simulink model "QD2_MissionCtrl_Swarm_4x_R2021a"  (R2021a)
settings: Solver=ode2  StartTime=0.0  StopTime=inf  FixedStep=0.001  RelTol=1e-3  EnableMultiTasking=on
undefined symbols (not defined in the file): datetime, Host, localhost, m, qc_get_step_size, saved_data
libraries: quarc_library x48, simulink x13, simulink_extras x1
(part 1 of 2)
settings Model: SimulationMode=external  ExtModeTrigDuration=10000  Creator=Admin  LastModifiedBy=jpineros
settings SolverCC: AlgebraicLoopSolver=TrustRegion  PositivePriorityOrder=on
settings DataIOCC: ReturnWorkspaceOutputs=off
settings DebuggingCC: SFUnexpectedBacktrackingDiag=warning  SFNoUnconditionalDefaultTransitionDiag=warning  SFExecutionAtInitializationDiag=none  ArithmeticOperatorsInVariantConditions=warning
settings SFSimCC: SimUseLocalCustomCode=off  CustomCodeUndefinedFunction=UseInterfaceOnly
settings RTWCC: Description=QUARC Win64 Target Using Toolchain  SystemTargetFile=quarc_win64.tlc  TemplateMakefile=quarc_default_tmf  RTWUseLocalCustomCode=off  Toolchain=QUARC win64 | nmake (64-bit Windows)  BuildConfiguration=Faster Runs  DLArmComputeVersion=20.02.1
settings CodeAppCC: StateflowObjectComments=on
settings STFCustomTargetCC: ConcurrentExecutionCompliant=on  SystemTargetFile=quarc_win64.tlc
settings GRTTargetCC: TargetLangStandard=C89/C90 (ANSI)  ParMdlRefBuildCompliant=off  CompOptLevelCompliant=off  CombineOutputUpdateFcns=off  MatFileLogging=off  CPPClassGenCompliant=off  GRTInterface=on  ExtMode=on  ExtModeMexFile=quarc_comm  ExtModeMexArgs='-w -d %d -uri %u -URI_Host_V1 tcpip://localhost:18001 -URI_Host_V2 tcpip://localhost:18002 -URI_Host_V3 tcpip://localhost:18003 -URI_Host_V4 tcpip://localhost:18004'
settings ConfigComp: CovMetricSettings=dw  CovSaveCumulativeToWorkspaceVar=on  CovSaveSingleToWorkspaceVar=on  CovExternalEMLEnable=off

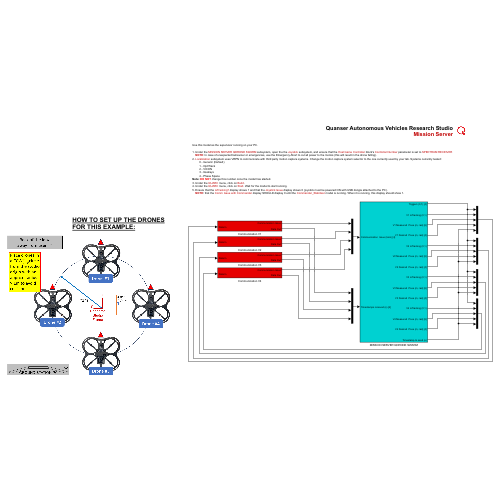
[thumbnail: Simulink's stored preview of the top-level diagram]
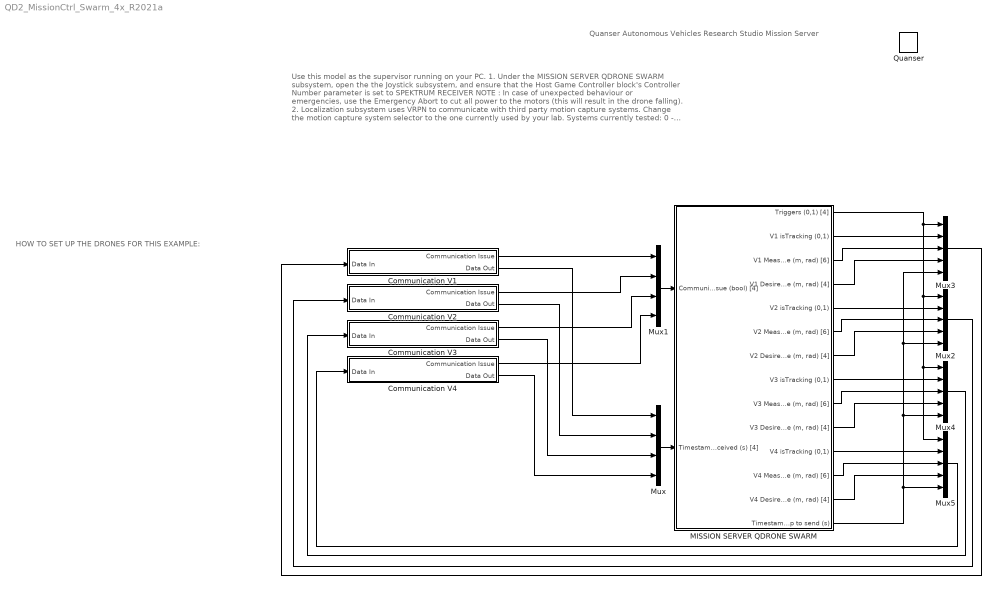
== system QD2_MissionCtrl_Swarm_4x_R2021a ==
  note: Use this model as the supervisor running on your PC.
      |
      | 1. Under the MISSION SERVER QDRONE SWARM subsystem, open the the Joystick subsystem, and ensure that the Host Game Controller block's Controller Number parameter is set to SPEKTRUM RECEIVER
      | NOTE : In case of unexpected behaviour or emergencies, use the Emergency Abort to cut all power to the motors (this will result in the drone falling).
      | 2. Localization subsystem uses VRPN to communicate with third party motion capture systems. Change the motion capture system selector to the one currently used by your lab. Systems currently tested:
      | 0 - Generic (Default)
      | 1 - OptiTrack
      | 2 - VICON
      | 3 - Qualisys
      | 4 - Phase Space
      | Note: DO NOT change this number once the model has started.
      | 3. Under the QUARC menu, click on Build .
      | 4. Under the QUARC menu, click on Start . Wait for the model to start running.
      | 5. Ensure that the isTracking? display shows 1 and that the Joystick Issue display shows 0 (joystick must be powered ON with USB dongle attached to the PC).
      | NOTE : that the Comm Issue with Commander display SHOULD display 0 until the Commander_Stabilizer model is running. When it is running, this display should show 1.
  note: Quanser Autonomous Vehicles Research Studio
      | Mission Server
  note: HOW TO SET UP THE DRONES FOR THIS EXAMPLE:
  Communication V1 : Subsystem
  Communication V2 : Subsystem
  Communication V3 : Subsystem
  Communication V4 : Subsystem
  MISSION SERVER QDRONE SWARM : Subsystem
  Mux : Mux
  Mux1 : Mux
  Mux{2..5} (4 alike) : Mux  Inputs=5
  Quanser : quarc_library/Logos/Quanser
  wires:
  Communication V1/1(Communication Issue) -> Mux1/1
  Communication V2/1(Communication Issue) -> Mux1/2
  Communication V3/1(Communication Issue) -> Mux1/3
  Communication V4/1(Communication Issue) -> Mux1/4
  Communication V4/2(Data Out) -> Mux/4
  Communication V3/2(Data Out) -> Mux/3
  Communication V2/2(Data Out) -> Mux/2
  Communication V1/2(Data Out) -> Mux/1
  MISSION SERVER QDRONE SWARM/14(Timestamp to send (s)) -> Mux5/5, Mux3/5, Mux2/5, Mux4/5
  Mux3/1 -> Communication V1/1(Data In)
  Mux2/1 -> Communication V2/1(Data In)
  Mux4/1 -> Communication V3/1(Data In)
  Mux5/1 -> Communication V4/1(Data In)
  Mux1/1 -> MISSION SERVER QDRONE SWARM/1(Communication Issue (bool) [4])
  Mux/1 -> MISSION SERVER QDRONE SWARM/2(Timestamps received (s) [4])
  MISSION SERVER QDRONE SWARM/3("V1 Measured Pose (m, rad) [6]") -> Mux3/3
  MISSION SERVER QDRONE SWARM/4("V1 Desired Pose (m, rad) [4]") -> Mux3/4
  MISSION SERVER QDRONE SWARM/6("V2 Measured Pose (m, rad) [6]") -> Mux2/3
  MISSION SERVER QDRONE SWARM/7("V2 Desired Pose (m, rad) [4]") -> Mux2/4
  MISSION SERVER QDRONE SWARM/9("V3 Measured Pose (m, rad) [6]") -> Mux4/3
  MISSION SERVER QDRONE SWARM/10("V3 Desired Pose (m, rad) [4]") -> Mux4/4
  MISSION SERVER QDRONE SWARM/12("V4 Measured Pose (m, rad) [6]") -> Mux5/3
  MISSION SERVER QDRONE SWARM/13("V4 Desired Pose (m, rad) [4]") -> Mux5/4
  MISSION SERVER QDRONE SWARM/1(Triggers (0,1) [4]) -> Mux5/1, Mux4/1, Mux2/1, Mux3/1
  MISSION SERVER QDRONE SWARM/2(V1 isTracking (0,1)) -> Mux3/2
  MISSION SERVER QDRONE SWARM/5(V2 isTracking (0,1)) -> Mux2/2
  MISSION SERVER QDRONE SWARM/8(V3 isTracking (0,1)) -> Mux4/2
  MISSION SERVER QDRONE SWARM/11(V4 isTracking (0,1)) -> Mux5/2

== system QD2_MissionCtrl_Swarm_4x_R2021a/Communication V1 ==
  note: Argument (-URI_Host_V1) is set at the MEX-file arguments
      | found at Model Configuration Properties > Code Generation > Interface
      |
      | Format:
      | tcpip://localhost:18001
  Data In : Inport
  Constant : Constant
  Detect Communication loss : Subsystem
  Model Argument : quarc_library/Sources/Signals/Model Argument  argument_name=URI_Host_V1  has_value=on  data_type_mode=Specify via dialog  data_type=char  max_length=80  default_value=0  default_string=tcpip://localhost:18001  variable_size=off
      settings: AttributesFormatString=(-%<argument_name>)  SourceProductName=QUARC Targets
  Stream Server : quarc_library/Communications/Basic/Stream Server  uri_source=External input port  uri=tcpip://localhost:18877  send_buffer_size=1460  receive_buffer_size=1460  byte_order=little endian (Intel - LSB first)  optimization=Minimum latency  send_options=Send most recent data  receive_options=Receive most recent data  default_value=zeros(1,1)  sample_time=qc_get_step_size  active=off  implementation=Use blocking I/O in a separate thread  send_fifo_size=1000  receive_fifo_size=1000  send_priority=0  receive_priority=0  send_dimensions=off  receive_dimensions=off  max_dimensions=-1  data_type=Inherited via back propagation  type_expr=BusObject
  "String Display " : quarc_library/Strings/String Display  alignment=center  display_mode=Single line  sample_time=-1  use_new=off
      settings: SourceProductName=QUARC Targets
  Terminator1 : Terminator
  Terminator2 : Terminator
  Communication Issue : Outport  VectorParamsAs1DForOutWhenUnconnected=off
  Data Out : Outport  Port=2  VectorParamsAs1DForOutWhenUnconnected=off
  wires:
  Detect Communication loss/1(Communication Issue (0,1)) -> Communication Issue/1
  Stream Server/1 -> Detect Communication loss/1(State)
  Stream Server/2 -> Detect Communication loss/2(Error)
  Stream Server/4 -> Data Out/1
  Model Argument/1 -> Stream Server/3, "String Display "/1
  Stream Server/5 -> Terminator1/1
  Stream Server/3 -> Terminator2/1
  Data In/1 -> Stream Server/1
  Constant/1 -> Stream Server/2

== system QD2_MissionCtrl_Swarm_4x_R2021a/Communication V2 ==
  note: Argument (-URI_Host_V2) is set at the MEX-file arguments
      | found at Model Configuration Properties > Code Generation > Interface
      |
      | Format:
      | tcpip://localhost:18002
  Data In : Inport
  Constant : Constant
  Detect Communication loss : Subsystem
  Model Argument : quarc_library/Sources/Signals/Model Argument  argument_name=URI_Host_V2  has_value=on  data_type_mode=Specify via dialog  data_type=char  max_length=80  default_value=0  default_string=tcpip://localhost:18002  variable_size=off
      settings: AttributesFormatString=(-%<argument_name>)  SourceProductName=QUARC Targets
  Stream Server : quarc_library/Communications/Basic/Stream Server  uri_source=External input port  uri=tcpip://localhost:18877  send_buffer_size=1460  receive_buffer_size=1460  byte_order=little endian (Intel - LSB first)  optimization=Minimum latency  send_options=Send most recent data  receive_options=Receive most recent data  default_value=zeros(1,1)  sample_time=qc_get_step_size  active=off  implementation=Use blocking I/O in a separate thread  send_fifo_size=1000  receive_fifo_size=1000  send_priority=0  receive_priority=0  send_dimensions=off  receive_dimensions=off  max_dimensions=-1  data_type=Inherited via back propagation  type_expr=BusObject
  "String Display " : quarc_library/Strings/String Display  alignment=center  display_mode=Single line  sample_time=-1  use_new=off
      settings: SourceProductName=QUARC Targets
  Terminator1 : Terminator
  Terminator2 : Terminator
  Communication Issue : Outport  VectorParamsAs1DForOutWhenUnconnected=off
  Data Out : Outport  Port=2  VectorParamsAs1DForOutWhenUnconnected=off
  wires:
  Constant/1 -> Stream Server/2
  Data In/1 -> Stream Server/1
  Stream Server/3 -> Terminator2/1
  Stream Server/5 -> Terminator1/1
  Model Argument/1 -> "String Display "/1, Stream Server/3
  Stream Server/4 -> Data Out/1
  Stream Server/2 -> Detect Communication loss/2(Error)
  Stream Server/1 -> Detect Communication loss/1(State)
  Detect Communication loss/1(Communication Issue (0,1)) -> Communication Issue/1

== system QD2_MissionCtrl_Swarm_4x_R2021a/Communication V3 ==
  note: Argument (-URI_Host_V3) is set at the MEX-file arguments
      | found at Model Configuration Properties > Code Generation > Interface
      |
      | Format:
      | tcpip://localhost:18003
  Data In : Inport
  Constant : Constant
  Detect Communication loss : Subsystem
  Model Argument : quarc_library/Sources/Signals/Model Argument  argument_name=URI_Host_V3  has_value=on  data_type_mode=Specify via dialog  data_type=char  max_length=80  default_value=0  default_string=tcpip://localhost:18003  variable_size=off
      settings: AttributesFormatString=(-%<argument_name>)  SourceProductName=QUARC Targets
  Stream Server : quarc_library/Communications/Basic/Stream Server  uri_source=External input port  uri=tcpip://localhost:18877  send_buffer_size=1460  receive_buffer_size=1460  byte_order=little endian (Intel - LSB first)  optimization=Minimum latency  send_options=Send most recent data  receive_options=Receive most recent data  default_value=zeros(1,1)  sample_time=qc_get_step_size  active=off  implementation=Use blocking I/O in a separate thread  send_fifo_size=1000  receive_fifo_size=1000  send_priority=0  receive_priority=0  send_dimensions=off  receive_dimensions=off  max_dimensions=-1  data_type=Inherited via back propagation  type_expr=BusObject
  "String Display " : quarc_library/Strings/String Display  alignment=center  display_mode=Single line  sample_time=-1  use_new=off
      settings: SourceProductName=QUARC Targets
  Terminator1 : Terminator
  Terminator2 : Terminator
  Communication Issue : Outport  VectorParamsAs1DForOutWhenUnconnected=off
  Data Out : Outport  Port=2  VectorParamsAs1DForOutWhenUnconnected=off
  wires:
  Detect Communication loss/1(Communication Issue (0,1)) -> Communication Issue/1
  Stream Server/1 -> Detect Communication loss/1(State)
  Stream Server/2 -> Detect Communication loss/2(Error)
  Stream Server/4 -> Data Out/1
  Model Argument/1 -> Stream Server/3, "String Display "/1
  Stream Server/5 -> Terminator1/1
  Stream Server/3 -> Terminator2/1
  Data In/1 -> Stream Server/1
  Constant/1 -> Stream Server/2

== system QD2_MissionCtrl_Swarm_4x_R2021a/Communication V4 ==
  note: Argument (-URI_Host_V4) is set at the MEX-file arguments
      | found at Model Configuration Properties > Code Generation > Interface
      |
      | Format:
      | tcpip://localhost:18004
  Data In : Inport
  Constant : Constant
  Detect Communication loss : Subsystem
  Model Argument : quarc_library/Sources/Signals/Model Argument  argument_name=URI_Host_V4  has_value=on  data_type_mode=Specify via dialog  data_type=char  max_length=80  default_value=0  default_string=tcpip://localhost:18004  variable_size=off
      settings: AttributesFormatString=(-%<argument_name>)  SourceProductName=QUARC Targets
  Stream Server : quarc_library/Communications/Basic/Stream Server  uri_source=External input port  uri=tcpip://localhost:18877  send_buffer_size=1460  receive_buffer_size=1460  byte_order=little endian (Intel - LSB first)  optimization=Minimum latency  send_options=Send most recent data  receive_options=Receive most recent data  default_value=zeros(1,1)  sample_time=qc_get_step_size  active=off  implementation=Use blocking I/O in a separate thread  send_fifo_size=1000  receive_fifo_size=1000  send_priority=0  receive_priority=0  send_dimensions=off  receive_dimensions=off  max_dimensions=-1  data_type=Inherited via back propagation  type_expr=BusObject
  "String Display " : quarc_library/Strings/String Display  alignment=center  display_mode=Single line  sample_time=-1  use_new=off
      settings: SourceProductName=QUARC Targets
  Terminator1 : Terminator
  Terminator2 : Terminator
  Communication Issue : Outport  VectorParamsAs1DForOutWhenUnconnected=off
  Data Out : Outport  Port=2  VectorParamsAs1DForOutWhenUnconnected=off
  wires:
  Constant/1 -> Stream Server/2
  Data In/1 -> Stream Server/1
  Stream Server/3 -> Terminator2/1
  Stream Server/5 -> Terminator1/1
  Model Argument/1 -> "String Display "/1, Stream Server/3
  Stream Server/4 -> Data Out/1
  Stream Server/2 -> Detect Communication loss/2(Error)
  Stream Server/1 -> Detect Communication loss/1(State)
  Detect Communication loss/1(Communication Issue (0,1)) -> Communication Issue/1

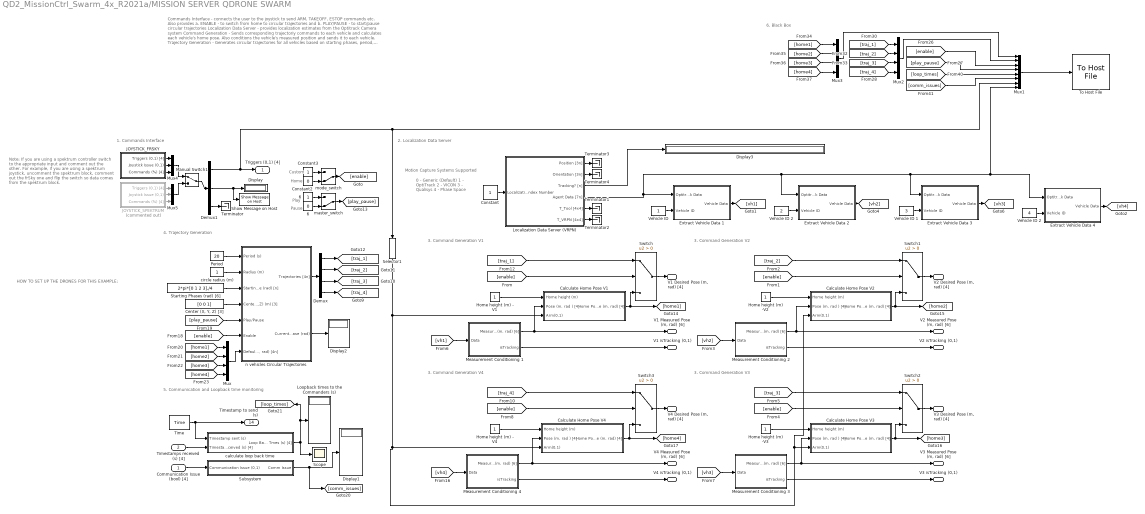
== system QD2_MissionCtrl_Swarm_4x_R2021a/MISSION SERVER QDRONE SWARM ==
  note: Commands Interface - connects the user to the joystick to send ARM, TAKEOFF, ESTOP commands etc. Also provides
      | a. ENABLE - to switch from home to circular trajectories and
      | b. PLAY/PAUSE - to start/pause circular trajectories
      | Localization Data Server - provides localization estimates from the Optitrack Camera system
      | Command Generation - Sends corresponding trajectoriy commands to each vehicle and calculates each vehicle's home pose. Also conditions the vehicle's measured position and sends it to each vehicle.
      | Trajectory Generation - Generates circular trajectories for all vehicles based on starting phases, period, radus and center location. When ENABLE is low, it switches to the trajectory at the Default (m, rad) [4] input
      | Communication and Loopback time monitoring - monitors communication issues with any vehicle, and also displays the loopback time to each model (time taken to send a packet to a vehicle and receive it back immediately).
      | Black Box: Logs selected data into log file for offline review and analysis.
  note: 6. Black Box
  note: 5. Communication and Loopback time monitoring
  note: 4. Trajectory Generation
  note: 2. Localization Data Server
  note: 1. Commands Interface
  note: Home
  note: Custom
  note: 3. Command Generation V1
  note: 3. Command Generation V2
  note: 3. Command Generation V3
  note: 3. Command Generation V4
  note: Pause
  note: Play
  note: HOW TO SET UP THE DRONES FOR THIS EXAMPLE:
  note: Note:
      | If you are using a spektrum controller switch to the appropriate input and comment out the other.
      | For example, if you are using a spektrum joystick, uncomment the spektrum block, comment out the frSky one and flip the switch so data comes from the spektrum block.
  note: Motion Capture Systems Supported
  note: 0 - Generic (Default)
      | 1 - OptiTrack
      | 2 - VICON
      | 3 - Qualisys
      | 4 - Phase Space
  Communication Issue (bool) [4] : Inport
  Timestamps received (s) [4] : Inport  Port=2
  "          6" : Constant
  "   6" : Constant  Value=0
  Calculate Home Pose V1 : Subsystem
  Calculate Home Pose V2 : Subsystem
  Calculate Home Pose V3 : Subsystem
  Calculate Home Pose V4 : Subsystem
  "Center (X, Y, Z) [3]" : Constant  Value=[0 0 1]
  Constant : Constant
  Constant2 : Constant  Value=0
  Constant3 : Constant
  Demux : Demux  Outputs=[4 4 4 4 ]
  Demux1 : Demux  Outputs=[4 1 4]
  Display{,1..3} (4 alike) : Display
  Extract Vehicle Data 1 : Subsystem
  Extract Vehicle Data 2 : Subsystem
  Extract Vehicle Data 3 : Subsystem
  Extract Vehicle Data 4 : Subsystem
  Home height (m) - V1 : Constant
  Home height (m) - V4 : Constant
  Home height (m) -V2 : Constant
  Home height (m) -V3 : Constant
  JOYSTICK_FRSKY : Subsystem
      mask Display: image('$imagefile'); % Use "Edit Image" on toolstrip to change.
  JOYSTICK_SPEKTRUM : Subsystem  Commented=on
      mask Display: image('$imagefile'); % Use "Edit Image" on toolstrip to change.
  "Localization Data Server (VRPN) " : Subsystem
  Loopback times to the Commanders (s) : Display
  Manual Switch1 : ManualSwitch
  Measurement Conditioning 1 : Subsystem
  Measurement Conditioning 2 : Subsystem
  Measurement Conditioning 3 : Subsystem
  Measurement Conditioning 4 : Subsystem
  Mux : Mux
  Mux1 : Mux  Inputs=8
  Mux2 : Mux
  Mux3 : Mux
  Mux4 : Mux  Inputs=[4 1 4]
  Mux5 : Mux  Inputs=[4 1 4]
  Period : Constant  Value=20
  Scope : Scope
  Selector1 : Selector  InputPortWidth=4  IndexOptions=Index vector (dialog)  Indices=[1]  OutputSizes=1
  "Show Message on Host " : quarc_library/Sinks/Error Handling/Show Message on Host  message_type=Fixed error message  message_icon=Warning  message=Mission Server: Joystick Disconnected
      settings: AttributesFormatString="\"%<message>\""  SourceProductName=QUARC Targets
  Starting Phases (rad) [6] : Constant  Value=2*pi*[0 1 2 3]./4
  Subsystem : Subsystem
  Switch{,1..3} (4 alike) : Switch  Criteria=u2 > Threshold
  Terminator{,1..4} (5 alike) : Terminator
  Time : quarc_library/Sources/Time/Time  time_source=Wall clock  sample_time=qc_get_step_size
  To Host File : quarc_library/Sinks/To Host/To Host File  source=Specify via dialog (do not evaluate)  file_name=saved_data/%m/%{char(datetime)}.mat  variable_name=data  decimation=1  sample_time=-1  file_format=MAT-file v.4  options=No header or footer  append=off  final_file_name=saved_data/QD2_MissionCtrl_Swarm_4x_R2021a_/2025-05-01 15-23-55.mat  bitrate=2000000
  Vehicle ID : Constant
  Vehicle ID 1 : Constant  Value=3
  Vehicle ID 2 : Constant  Value=4
  "Vehicle ID 2 " : Constant  Value=2
  calculate loop back time : Subsystem
  circle radius (m) : Constant
  master_switch : ManualSwitch  CurrentSetting=0
  mode_switch : ManualSwitch  CurrentSetting=0
  n vehicles Circular Trajectories : Subsystem
  Triggers (0,1) [4] : Outport  VectorParamsAs1DForOutWhenUnconnected=off
  V1 isTracking (0,1) : Outport  Port=2  VectorParamsAs1DForOutWhenUnconnected=off
  "V1 Measured Pose (m, rad) [6]" : Outport  Port=3  VectorParamsAs1DForOutWhenUnconnected=off
  "V1 Desired Pose (m, rad) [4]" : Outport  Port=4  VectorParamsAs1DForOutWhenUnconnected=off
  V2 isTracking (0,1) : Outport  Port=5  VectorParamsAs1DForOutWhenUnconnected=off
  "V2 Measured Pose (m, rad) [6]" : Outport  Port=6  VectorParamsAs1DForOutWhenUnconnected=off
  "V2 Desired Pose (m, rad) [4]" : Outport  Port=7  VectorParamsAs1DForOutWhenUnconnected=off
  V3 isTracking (0,1) : Outport  Port=8  VectorParamsAs1DForOutWhenUnconnected=off
  "V3 Measured Pose (m, rad) [6]" : Outport  Port=9  VectorParamsAs1DForOutWhenUnconnected=off
  "V3 Desired Pose (m, rad) [4]" : Outport  Port=10  VectorParamsAs1DForOutWhenUnconnected=off
  V4 isTracking (0,1) : Outport  Port=11  VectorParamsAs1DForOutWhenUnconnected=off
  "V4 Measured Pose (m, rad) [6]" : Outport  Port=12  VectorParamsAs1DForOutWhenUnconnected=off
  "V4 Desired Pose (m, rad) [4]" : Outport  Port=13  VectorParamsAs1DForOutWhenUnconnected=off
  Timestamp to send (s) : Outport  Port=14  VectorParamsAs1DForOutWhenUnconnected=off
  wires:
  Demux1/2 -> Display/1, "Show Message on Host "/1
  Constant3/1 -> mode_switch/1
  Constant2/1 -> mode_switch/2
  Demux1/3 -> Terminator/1
  "   6"/1 -> master_switch/2
  Period/1 -> n vehicles Circular Trajectories/1(Period (s))
  circle radius (m)/1 -> n vehicles Circular Trajectories/2(Radius (m))
  "          6"/1 -> master_switch/1
  [play_pause] -> n vehicles Circular Trajectories/5(Play/Pause)
  Demux1/1 -> Triggers (0,1) [4]/1, Selector1/1, Mux1/7
  Time/1 -> Timestamp to send (s)/1, calculate loop back time/1(Timestamp sent (s))
  Timestamps received (s) [4]/1 -> calculate loop back time/2(Timestamps received (s) [4])
  Starting Phases (rad) [6]/1 -> n vehicles Circular Trajectories/3(Starting Phase (rad) [n])
  "Center (X, Y, Z) [3]"/1 -> n vehicles Circular Trajectories/4(Center (X,Y,Z) (m) [3])
  n vehicles Circular Trajectories/2(Current Phase (rad)) -> Display2/1
  Vehicle ID 1/1 -> Extract Vehicle Data 3/2(Vehicle ID)
  "Vehicle ID 2 "/1 -> Extract Vehicle Data 2/2(Vehicle ID)
  Vehicle ID/1 -> Extract Vehicle Data 1/2(Vehicle ID)
  Vehicle ID 2/1 -> Extract Vehicle Data 4/2(Vehicle ID)
  Measurement Conditioning 1/2(isTracking) -> V1 isTracking (0,1)/1
  Calculate Home Pose V1/1("Home Pose (m, rad) [4]") -> [home1], Switch/3
  [traj_1] -> Switch/1
  Home height (m) - V1/1 -> Calculate Home Pose V1/1(Home height (m))
  Measurement Conditioning 1/1("Measured Pose (m, rad) [6]") -> Calculate Home Pose V1/2("Pose (m, rad ) [4]"), "V1 Measured Pose (m, rad) [6]"/1
  Switch/1 -> "V1 Desired Pose (m, rad) [4]"/1
  mode_switch/1 -> [enable]
  [enable] -> Switch/2
  Extract Vehicle Data 1/1(Vehicle Data) -> [vh1]
  Extract Vehicle Data 4/1(Vehicle Data) -> [vh4]
  Extract Vehicle Data 2/1(Vehicle Data) -> [vh2]
  Extract Vehicle Data 3/1(Vehicle Data) -> [vh3]
  [vh1] -> Measurement Conditioning 1/1(Data)
  n vehicles Circular Trajectories/1(Trajectories [4n]) -> Demux/1
  Demux/1 -> [traj_1]
  Demux/2 -> [traj_2]
  Demux/3 -> [traj_3]
  Demux/4 -> [traj_4]
  [vh2] -> Measurement Conditioning 2/1(Data)
  [enable] -> Switch1/2
  Switch1/1 -> "V2 Desired Pose (m, rad) [4]"/1
  Measurement Conditioning 2/1("Measured Pose (m, rad) [6]") -> Calculate Home Pose V2/2("Pose (m, rad ) [4]"), "V2 Measured Pose (m, rad) [6]"/1
  Home height (m) -V2/1 -> Calculate Home Pose V2/1(Home height (m))
  [traj_2] -> Switch1/1
  Calculate Home Pose V2/1("Home Pose (m, rad) [4]") -> Switch1/3, [home2]
  Measurement Conditioning 2/2(isTracking) -> V2 isTracking (0,1)/1
  Measurement Conditioning 3/2(isTracking) -> V3 isTracking (0,1)/1
  Calculate Home Pose V3/1("Home Pose (m, rad) [4]") -> [home3], Switch2/3
  [traj_3] -> Switch2/1
  Home height (m) -V3/1 -> Calculate Home Pose V3/1(Home height (m))
  Measurement Conditioning 3/1("Measured Pose (m, rad) [6]") -> Calculate Home Pose V3/2("Pose (m, rad ) [4]"), "V3 Measured Pose (m, rad) [6]"/1
  Switch2/1 -> "V3 Desired Pose (m, rad) [4]"/1
  [enable] -> Switch2/2
  [vh3] -> Measurement Conditioning 3/1(Data)
  [vh4] -> Measurement Conditioning 4/1(Data)
  [enable] -> Switch3/2
  Switch3/1 -> "V4 Desired Pose (m, rad) [4]"/1
  Measurement Conditioning 4/1("Measured Pose (m, rad) [6]") -> Calculate Home Pose V4/2("Pose (m, rad ) [4]"), "V4 Measured Pose (m, rad) [6]"/1
  Home height (m) - V4/1 -> Calculate Home Pose V4/1(Home height (m))
  [traj_4] -> Switch3/1
  Calculate Home Pose V4/1("Home Pose (m, rad) [4]") -> [home4], Switch3/3
  Measurement Conditioning 4/2(isTracking) -> V4 isTracking (0,1)/1
  [enable] -> n vehicles Circular Trajectories/6(Enable)
  master_switch/1 -> [play_pause]
  Communication Issue (bool) [4]/1 -> Subsystem/1(Communication Issue (0,1))
  calculate loop back time/1(Loop Back Tmes (s) [4]) -> Scope/1, Loopback times to the Commanders (s)/1, [loop_times]
  Mux/1 -> n vehicles Circular Trajectories/7("Default (m, rad) [4n]")
  [home2] -> Mux/2
  [home3] -> Mux/3
  [home4] -> Mux/4
  [home1] -> Mux/1
  Mux1/1 -> To Host File/1
  [play_pause] -> Mux1/4
  [enable] -> Mux1/3
  Mux2/1 -> Mux1/2
  [home1] -> Mux3/1
  [home4] -> Mux3/4
  [home3] -> Mux3/3
  [home2] -> Mux3/2
  [traj_4] -> Mux2/4
  [traj_3] -> Mux2/3
  [traj_2] -> Mux2/2
  [traj_1] -> Mux2/1
  Mux3/1 -> Mux1/1
  Subsystem/1(Comm Issue) -> [comm_issues], Display1/1
  [comm_issues] -> Mux1/6
  [loop_times] -> Mux1/5
  "Localization Data Server (VRPN) "/4(Agent Data [7n]) -> Extract Vehicle Data 2/1(Optitrack Data), Extract Vehicle Data 3/1(Optitrack Data), Extract Vehicle Data 4/1(Optitrack Data), Mux1/8, Extract Vehicle Data 1/1(Optitrack Data)
  Selector1/1 -> Calculate Home Pose V1/3(Arm(0,1)), Calculate Home Pose V3/3(Arm(0,1)), Calculate Home Pose V2/3(Arm(0,1)), Calculate Home Pose V4/3(Arm(0,1))
  Mux4/1 -> Manual Switch1/1
  JOYSTICK_SPEKTRUM/1(Triggers (0,1) [4]) -> Mux5/1
  JOYSTICK_SPEKTRUM/3(Commands (%) [4]) -> Mux5/3
  JOYSTICK_FRSKY/3(Commands (%) [4]) -> Mux4/3
  JOYSTICK_SPEKTRUM/2(Joystick Issue (0,1)) -> Mux5/2
  Manual Switch1/1 -> Demux1/1
  Mux5/1 -> Manual Switch1/2
  JOYSTICK_FRSKY/2(Joystick Issue (0,1)) -> Mux4/2
  JOYSTICK_FRSKY/1(Triggers (0,1) [4]) -> Mux4/1
  Constant/1 -> "Localization Data Server (VRPN) "/1(Localization System Index Number)
  "Localization Data Server (VRPN) "/3(Tracking? [n]) -> Display3/1
  "Localization Data Server (VRPN) "/5(T_Tool [4x4]) -> Terminator1/1
  "Localization Data Server (VRPN) "/6(T_VRPN [4x4]) -> Terminator2/1
  "Localization Data Server (VRPN) "/1(Position [3n]) -> Terminator3/1
  "Localization Data Server (VRPN) "/2(Orientation [3n]) -> Terminator4/1

== system QD2_MissionCtrl_Swarm_4x_R2021a/Communication V1/Detect Communication loss ==
  State : Inport
  Error : Inport  Port=2
  Data Type Conversion : DataTypeConversion
  MATLAB Function : MATLAB Function  TreatAsAtomicUnit=on
  Terminator2 : Terminator
  Threshold : quarc_library/Discontinuities/Threshold  operator=>=  param_src=Specify via dialog  threshold=0.5  duration=0.1
      settings: SourceProductName=QUARC Targets
  Time : quarc_library/Sources/Time/Time  time_source=Wall clock  sample_time=qc_get_step_size
  Communication Issue (0,1) : Outport  VectorParamsAs1DForOutWhenUnconnected=off
  wires:
  Threshold/1 -> Data Type Conversion/1
  Data Type Conversion/1 -> Communication Issue (0,1)/1
  Threshold/2 -> Terminator2/1
  Time/1 -> MATLAB Function/1(time)
  State/1 -> MATLAB Function/2(state)
  MATLAB Function/1(stream_connection_loss) -> Threshold/1
  Error/1 -> MATLAB Function/3(error)

== system QD2_MissionCtrl_Swarm_4x_R2021a/Communication V2/Detect Communication loss ==
  State : Inport
  Error : Inport  Port=2
  Data Type Conversion : DataTypeConversion
  MATLAB Function : MATLAB Function  TreatAsAtomicUnit=on
  Terminator2 : Terminator
  Threshold : quarc_library/Discontinuities/Threshold  operator=>=  param_src=Specify via dialog  threshold=0.5  duration=0.1
      settings: SourceProductName=QUARC Targets
  Time : quarc_library/Sources/Time/Time  time_source=Wall clock  sample_time=qc_get_step_size
  Communication Issue (0,1) : Outport  VectorParamsAs1DForOutWhenUnconnected=off
  wires:
  Error/1 -> MATLAB Function/3(error)
  MATLAB Function/1(stream_connection_loss) -> Threshold/1
  State/1 -> MATLAB Function/2(state)
  Time/1 -> MATLAB Function/1(time)
  Threshold/2 -> Terminator2/1
  Data Type Conversion/1 -> Communication Issue (0,1)/1
  Threshold/1 -> Data Type Conversion/1

== system QD2_MissionCtrl_Swarm_4x_R2021a/Communication V3/Detect Communication loss ==
  State : Inport
  Error : Inport  Port=2
  Data Type Conversion : DataTypeConversion
  MATLAB Function : MATLAB Function  TreatAsAtomicUnit=on
  Terminator2 : Terminator
  Threshold : quarc_library/Discontinuities/Threshold  operator=>=  param_src=Specify via dialog  threshold=0.5  duration=0.1
      settings: SourceProductName=QUARC Targets
  Time : quarc_library/Sources/Time/Time  time_source=Wall clock  sample_time=qc_get_step_size
  Communication Issue (0,1) : Outport  VectorParamsAs1DForOutWhenUnconnected=off
  wires:
  Threshold/1 -> Data Type Conversion/1
  Data Type Conversion/1 -> Communication Issue (0,1)/1
  Threshold/2 -> Terminator2/1
  Time/1 -> MATLAB Function/1(time)
  State/1 -> MATLAB Function/2(state)
  MATLAB Function/1(stream_connection_loss) -> Threshold/1
  Error/1 -> MATLAB Function/3(error)

== system QD2_MissionCtrl_Swarm_4x_R2021a/Communication V4/Detect Communication loss ==
  State : Inport
  Error : Inport  Port=2
  Data Type Conversion : DataTypeConversion
  MATLAB Function : MATLAB Function  TreatAsAtomicUnit=on
  Terminator2 : Terminator
  Threshold : quarc_library/Discontinuities/Threshold  operator=>=  param_src=Specify via dialog  threshold=0.5  duration=0.1
      settings: SourceProductName=QUARC Targets
  Time : quarc_library/Sources/Time/Time  time_source=Wall clock  sample_time=qc_get_step_size
  Communication Issue (0,1) : Outport  VectorParamsAs1DForOutWhenUnconnected=off
  wires:
  Error/1 -> MATLAB Function/3(error)
  MATLAB Function/1(stream_connection_loss) -> Threshold/1
  State/1 -> MATLAB Function/2(state)
  Time/1 -> MATLAB Function/1(time)
  Threshold/2 -> Terminator2/1
  Data Type Conversion/1 -> Communication Issue (0,1)/1
  Threshold/1 -> Data Type Conversion/1

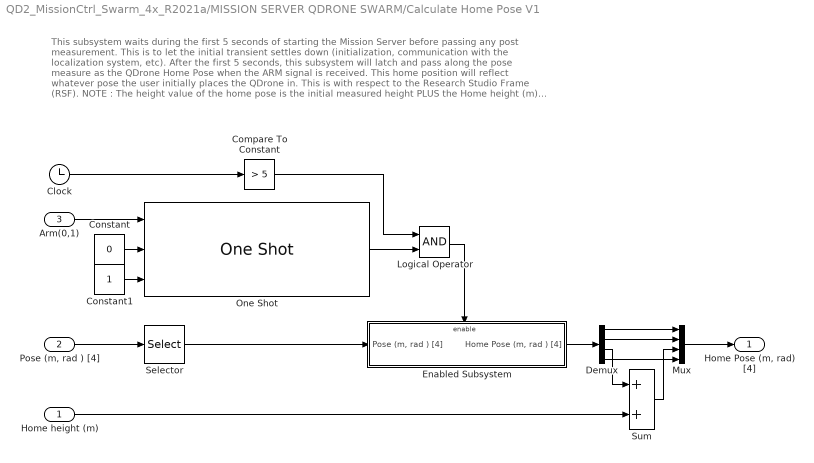
== system QD2_MissionCtrl_Swarm_4x_R2021a/MISSION SERVER QDRONE SWARM/Calculate Home Pose V1 ==
  note: This subsystem waits during the first 5 seconds of starting the Mission Server before passing any post measurement.
      | This is to let the initial transient settles down (initialization, communication with the localization system, etc).
      | After the first 5 seconds, this subsystem will latch and pass along the pose measure as the QDrone Home Pose when
      | the ARM signal is received.
      | This home position will reflect whatever pose the user initially places the QDrone in.
      | This is with respect to the Research Studio Frame (RSF).
      |
      | NOTE : The height value of the home pose is the initial measured height PLUS the Home height (m) input value.
  Home height (m) : Inport
  "Pose (m, rad ) [4]" : Inport  Port=2
  Arm(0,1) : Inport  Port=3
  Clock : Clock
  Compare To Constant : simulink/Logic and Bit Operations/Compare To Constant  relop=>  const=5  OutDataTypeStr=boolean
  Constant : Constant  Value=0
  Constant1 : Constant
  Demux : Demux
  Enabled Subsystem : Subsystem  TreatAsAtomicUnit=on
  Logical Operator : Logic  AllPortsSameDT=off  OutDataTypeStr=boolean
  Mux : Mux
  One Shot : quarc_library/Discontinuities/One Shot  trigger_type=Rising edge  redun_pulse=Ignore extraneous pulse  width_source=Specify via dialog  pulse_width=1/qc_get_step_size
      settings: SourceProductName=QUARC Targets
  Selector : Selector  InputPortWidth=6  IndexOptions=Index vector (dialog)  Indices=[1:3,6]  OutputSizes=1
  Sum : Sum
  "Home Pose (m, rad) [4]" : Outport  VectorParamsAs1DForOutWhenUnconnected=off
  wires:
  Constant/1 -> One Shot/2
  Constant1/1 -> One Shot/3
  Arm(0,1)/1 -> One Shot/1
  One Shot/1 -> Logical Operator/2
  "Pose (m, rad ) [4]"/1 -> Selector/1
  Clock/1 -> Compare To Constant/1
  Compare To Constant/1 -> Logical Operator/1
  Logical Operator/1 -> Enabled Subsystem/Enable
  Enabled Subsystem/1("Home Pose (m, rad ) [4]") -> Demux/1
  Demux/1 -> Mux/1
  Demux/2 -> Mux/2
  Demux/4 -> Mux/4
  Demux/3 -> Sum/1
  Sum/1 -> Mux/3
  Home height (m)/1 -> Sum/2
  Mux/1 -> "Home Pose (m, rad) [4]"/1
  Selector/1 -> Enabled Subsystem/1("Pose (m, rad ) [4] ")

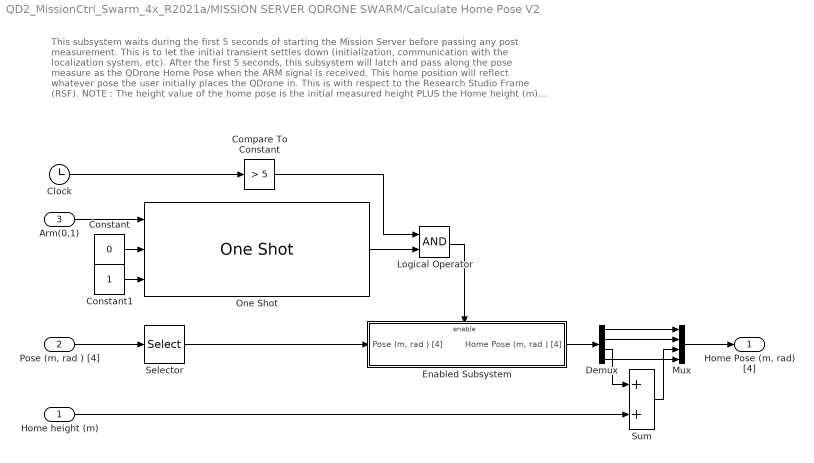
== system QD2_MissionCtrl_Swarm_4x_R2021a/MISSION SERVER QDRONE SWARM/Calculate Home Pose V2 ==
  note: This subsystem waits during the first 5 seconds of starting the Mission Server before passing any post measurement.
      | This is to let the initial transient settles down (initialization, communication with the localization system, etc).
      | After the first 5 seconds, this subsystem will latch and pass along the pose measure as the QDrone Home Pose when
      | the ARM signal is received.
      | This home position will reflect whatever pose the user initially places the QDrone in.
      | This is with respect to the Research Studio Frame (RSF).
      |
      | NOTE : The height value of the home pose is the initial measured height PLUS the Home height (m) input value.
  Home height (m) : Inport
  "Pose (m, rad ) [4]" : Inport  Port=2
  Arm(0,1) : Inport  Port=3
  Clock : Clock
  Compare To Constant : simulink/Logic and Bit Operations/Compare To Constant  relop=>  const=5  OutDataTypeStr=boolean
  Constant : Constant  Value=0
  Constant1 : Constant
  Demux : Demux
  Enabled Subsystem : Subsystem  TreatAsAtomicUnit=on
  Logical Operator : Logic  AllPortsSameDT=off  OutDataTypeStr=boolean
  Mux : Mux
  One Shot : quarc_library/Discontinuities/One Shot  trigger_type=Rising edge  redun_pulse=Ignore extraneous pulse  width_source=Specify via dialog  pulse_width=1/qc_get_step_size
      settings: SourceProductName=QUARC Targets
  Selector : Selector  InputPortWidth=6  IndexOptions=Index vector (dialog)  Indices=[1:3,6]  OutputSizes=1
  Sum : Sum
  "Home Pose (m, rad) [4]" : Outport  VectorParamsAs1DForOutWhenUnconnected=off
  wires:
  Constant/1 -> One Shot/2
  Constant1/1 -> One Shot/3
  Arm(0,1)/1 -> One Shot/1
  One Shot/1 -> Logical Operator/2
  "Pose (m, rad ) [4]"/1 -> Selector/1
  Clock/1 -> Compare To Constant/1
  Compare To Constant/1 -> Logical Operator/1
  Logical Operator/1 -> Enabled Subsystem/Enable
  Enabled Subsystem/1("Home Pose (m, rad ) [4]") -> Demux/1
  Demux/1 -> Mux/1
  Demux/2 -> Mux/2
  Demux/4 -> Mux/4
  Demux/3 -> Sum/1
  Sum/1 -> Mux/3
  Home height (m)/1 -> Sum/2
  Mux/1 -> "Home Pose (m, rad) [4]"/1
  Selector/1 -> Enabled Subsystem/1("Pose (m, rad ) [4] ")

== system QD2_MissionCtrl_Swarm_4x_R2021a/MISSION SERVER QDRONE SWARM/Calculate Home Pose V3 ==
  note: This subsystem waits during the first 5 seconds of starting the Mission Server before passing any post measurement.
      | This is to let the initial transient settles down (initialization, communication with the localization system, etc).
      | After the first 5 seconds, this subsystem will latch and pass along the pose measure as the QDrone Home Pose when
      | the ARM signal is received.
      | This home position will reflect whatever pose the user initially places the QDrone in.
      | This is with respect to the Research Studio Frame (RSF).
      |
      | NOTE : The height value of the home pose is the initial measured height PLUS the Home height (m) input value.
  Home height (m) : Inport
  "Pose (m, rad ) [4]" : Inport  Port=2
  Arm(0,1) : Inport  Port=3
  Clock : Clock
  Compare To Constant : simulink/Logic and Bit Operations/Compare To Constant  relop=>  const=5  OutDataTypeStr=boolean
  Constant : Constant  Value=0
  Constant1 : Constant
  Demux : Demux
  Enabled Subsystem : Subsystem  TreatAsAtomicUnit=on
  Logical Operator : Logic  AllPortsSameDT=off  OutDataTypeStr=boolean
  Mux : Mux
  One Shot : quarc_library/Discontinuities/One Shot  trigger_type=Rising edge  redun_pulse=Ignore extraneous pulse  width_source=Specify via dialog  pulse_width=1/qc_get_step_size
      settings: SourceProductName=QUARC Targets
  Selector : Selector  InputPortWidth=6  IndexOptions=Index vector (dialog)  Indices=[1:3,6]  OutputSizes=1
  Sum : Sum
  "Home Pose (m, rad) [4]" : Outport  VectorParamsAs1DForOutWhenUnconnected=off
  wires:
  Constant/1 -> One Shot/2
  Constant1/1 -> One Shot/3
  Arm(0,1)/1 -> One Shot/1
  One Shot/1 -> Logical Operator/2
  "Pose (m, rad ) [4]"/1 -> Selector/1
  Clock/1 -> Compare To Constant/1
  Compare To Constant/1 -> Logical Operator/1
  Logical Operator/1 -> Enabled Subsystem/Enable
  Enabled Subsystem/1("Home Pose (m, rad ) [4]") -> Demux/1
  Demux/1 -> Mux/1
  Demux/2 -> Mux/2
  Demux/4 -> Mux/4
  Demux/3 -> Sum/1
  Sum/1 -> Mux/3
  Home height (m)/1 -> Sum/2
  Mux/1 -> "Home Pose (m, rad) [4]"/1
  Selector/1 -> Enabled Subsystem/1("Pose (m, rad ) [4] ")

== system QD2_MissionCtrl_Swarm_4x_R2021a/MISSION SERVER QDRONE SWARM/Calculate Home Pose V4 ==
  note: This subsystem waits during the first 5 seconds of starting the Mission Server before passing any post measurement.
      | This is to let the initial transient settles down (initialization, communication with the localization system, etc).
      | After the first 5 seconds, this subsystem will latch and pass along the pose measure as the QDrone Home Pose when
      | the ARM signal is received.
      | This home position will reflect whatever pose the user initially places the QDrone in.
      | This is with respect to the Research Studio Frame (RSF).
      |
      | NOTE : The height value of the home pose is the initial measured height PLUS the Home height (m) input value.
  Home height (m) : Inport
  "Pose (m, rad ) [4]" : Inport  Port=2
  Arm(0,1) : Inport  Port=3
  Clock : Clock
  Compare To Constant : simulink/Logic and Bit Operations/Compare To Constant  relop=>  const=5  OutDataTypeStr=boolean
  Constant : Constant  Value=0
  Constant1 : Constant
  Demux : Demux
  Enabled Subsystem : Subsystem  TreatAsAtomicUnit=on
  Logical Operator : Logic  AllPortsSameDT=off  OutDataTypeStr=boolean
  Mux : Mux
  One Shot : quarc_library/Discontinuities/One Shot  trigger_type=Rising edge  redun_pulse=Ignore extraneous pulse  width_source=Specify via dialog  pulse_width=1/qc_get_step_size
      settings: SourceProductName=QUARC Targets
  Selector : Selector  InputPortWidth=6  IndexOptions=Index vector (dialog)  Indices=[1:3,6]  OutputSizes=1
  Sum : Sum
  "Home Pose (m, rad) [4]" : Outport  VectorParamsAs1DForOutWhenUnconnected=off
  wires:
  Constant/1 -> One Shot/2
  Constant1/1 -> One Shot/3
  Arm(0,1)/1 -> One Shot/1
  One Shot/1 -> Logical Operator/2
  "Pose (m, rad ) [4]"/1 -> Selector/1
  Clock/1 -> Compare To Constant/1
  Compare To Constant/1 -> Logical Operator/1
  Logical Operator/1 -> Enabled Subsystem/Enable
  Enabled Subsystem/1("Home Pose (m, rad ) [4]") -> Demux/1
  Demux/1 -> Mux/1
  Demux/2 -> Mux/2
  Demux/4 -> Mux/4
  Demux/3 -> Sum/1
  Sum/1 -> Mux/3
  Home height (m)/1 -> Sum/2
  Mux/1 -> "Home Pose (m, rad) [4]"/1
  Selector/1 -> Enabled Subsystem/1("Pose (m, rad ) [4] ")

== system QD2_MissionCtrl_Swarm_4x_R2021a/MISSION SERVER QDRONE SWARM/Extract Vehicle Data 1 ==
  Optitrack Data : Inport
  Vehicle ID : Inport  Port=2
  Data Type Conversion10 : DataTypeConversion
  Data Type Conversion11 : DataTypeConversion
  Data Type Conversion9 : DataTypeConversion
  Extract Object Data : MATLAB Function  TreatAsAtomicUnit=on
  Mux1 : Mux  Inputs=3
  Reshape : Reshape
  Reshape1 : Reshape
  Reshape2 : Reshape
  Vehicle Data : Outport  VectorParamsAs1DForOutWhenUnconnected=off
  wires:
  Reshape2/1 -> Data Type Conversion9/1
  Reshape1/1 -> Data Type Conversion10/1
  Reshape/1 -> Data Type Conversion11/1
  Data Type Conversion9/1 -> Mux1/3
  Data Type Conversion10/1 -> Mux1/2
  Data Type Conversion11/1 -> Mux1/1
  Extract Object Data/2(orientation) -> Reshape1/1
  Extract Object Data/3(tracking) -> Reshape2/1
  Extract Object Data/1(position) -> Reshape/1
  Mux1/1 -> Vehicle Data/1
  Optitrack Data/1 -> Extract Object Data/1(data)
  Vehicle ID/1 -> Extract Object Data/2(index)

== system QD2_MissionCtrl_Swarm_4x_R2021a/MISSION SERVER QDRONE SWARM/Extract Vehicle Data 2 ==
  Optitrack Data : Inport
  Vehicle ID : Inport  Port=2
  Data Type Conversion10 : DataTypeConversion
  Data Type Conversion11 : DataTypeConversion
  Data Type Conversion9 : DataTypeConversion
  Extract Object Data : MATLAB Function  TreatAsAtomicUnit=on
  Mux1 : Mux  Inputs=3
  Reshape : Reshape
  Reshape1 : Reshape
  Reshape2 : Reshape
  Vehicle Data : Outport  VectorParamsAs1DForOutWhenUnconnected=off
  wires:
  Vehicle ID/1 -> Extract Object Data/2(index)
  Optitrack Data/1 -> Extract Object Data/1(data)
  Mux1/1 -> Vehicle Data/1
  Extract Object Data/1(position) -> Reshape/1
  Extract Object Data/3(tracking) -> Reshape2/1
  Extract Object Data/2(orientation) -> Reshape1/1
  Data Type Conversion11/1 -> Mux1/1
  Data Type Conversion10/1 -> Mux1/2
  Data Type Conversion9/1 -> Mux1/3
  Reshape/1 -> Data Type Conversion11/1
  Reshape1/1 -> Data Type Conversion10/1
  Reshape2/1 -> Data Type Conversion9/1

== system QD2_MissionCtrl_Swarm_4x_R2021a/MISSION SERVER QDRONE SWARM/Extract Vehicle Data 3 ==
  Optitrack Data : Inport
  Vehicle ID : Inport  Port=2
  Data Type Conversion10 : DataTypeConversion
  Data Type Conversion11 : DataTypeConversion
  Data Type Conversion9 : DataTypeConversion
  Extract Object Data : MATLAB Function  TreatAsAtomicUnit=on
  Mux1 : Mux  Inputs=3
  Reshape : Reshape
  Reshape1 : Reshape
  Reshape2 : Reshape
  Vehicle Data : Outport  VectorParamsAs1DForOutWhenUnconnected=off
  wires:
  Vehicle ID/1 -> Extract Object Data/2(index)
  Optitrack Data/1 -> Extract Object Data/1(data)
  Mux1/1 -> Vehicle Data/1
  Extract Object Data/1(position) -> Reshape/1
  Extract Object Data/3(tracking) -> Reshape2/1
  Extract Object Data/2(orientation) -> Reshape1/1
  Data Type Conversion11/1 -> Mux1/1
  Data Type Conversion10/1 -> Mux1/2
  Data Type Conversion9/1 -> Mux1/3
  Reshape/1 -> Data Type Conversion11/1
  Reshape1/1 -> Data Type Conversion10/1
  Reshape2/1 -> Data Type Conversion9/1

== system QD2_MissionCtrl_Swarm_4x_R2021a/MISSION SERVER QDRONE SWARM/Extract Vehicle Data 4 ==
  Optitrack Data : Inport
  Vehicle ID : Inport  Port=2
  Data Type Conversion10 : DataTypeConversion
  Data Type Conversion11 : DataTypeConversion
  Data Type Conversion9 : DataTypeConversion
  Extract Object Data : MATLAB Function  TreatAsAtomicUnit=on
  Mux1 : Mux  Inputs=3
  Reshape : Reshape
  Reshape1 : Reshape
  Reshape2 : Reshape
  Vehicle Data : Outport  VectorParamsAs1DForOutWhenUnconnected=off
  wires:
  Reshape2/1 -> Data Type Conversion9/1
  Reshape1/1 -> Data Type Conversion10/1
  Reshape/1 -> Data Type Conversion11/1
  Data Type Conversion9/1 -> Mux1/3
  Data Type Conversion10/1 -> Mux1/2
  Data Type Conversion11/1 -> Mux1/1
  Extract Object Data/2(orientation) -> Reshape1/1
  Extract Object Data/3(tracking) -> Reshape2/1
  Extract Object Data/1(position) -> Reshape/1
  Mux1/1 -> Vehicle Data/1
  Optitrack Data/1 -> Extract Object Data/1(data)
  Vehicle ID/1 -> Extract Object Data/2(index)

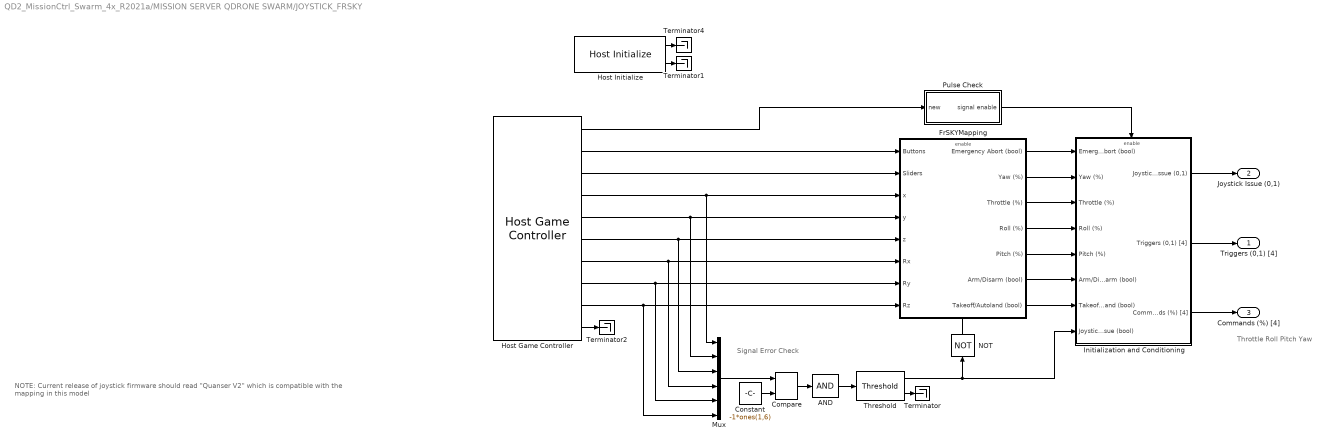
== system QD2_MissionCtrl_Swarm_4x_R2021a/MISSION SERVER QDRONE SWARM/JOYSTICK_FRSKY ==
  note: Throttle
      | Roll
      | Pitch
      | Yaw
  note: Signal Error Check
  note: NOTE: Current release of joystick firmware should read "Quanser V2" which is compatible with the mapping in this model
  AND : Logic  Inputs=1  AllPortsSameDT=off  OutDataTypeStr=boolean
  Compare : quarc_library/Logic Operations/Compare  operator===  output_data_type=boolean
      settings: SourceProductName=QUARC Targets
  Constant : Constant  Value=-1*ones(1,6)
  FrSKYMapping : Subsystem
  Host Game Controller : quarc_library/Devices/Peripherals/Host/Host Game Controller  object_name=Host-1  controller=1  buffer_size=20  deadzone=[]  saturation=[]  sample_time=qc_get_step_size  auto_center=off  enabled=on  debug_mode=off
      settings: SourceProductName=QUARC Targets
  Host Initialize : quarc_library/Devices/Peripherals/Host/Host Initialize  object_name=Host-1  uri_source=Use external mode communications  uri=tcpip://localhost:18001  send_buffer_size=1000  receive_buffer_size=1000  thread_priority=0  run_client=on  use_window=off  window_position=[]  sample_time=qc_get_step_size  active=on
      settings: SourceProductName=QUARC Targets
  Initialization and Conditioning : Subsystem  TreatAsAtomicUnit=on
  Mux : Mux  Inputs=6
  NOT : Logic  Operator=NOT  IconShape=distinctive  AllPortsSameDT=off  OutDataTypeStr=boolean
  Pulse Check : Subsystem  TreatAsAtomicUnit=on
  Terminator{,1..2,4} (4 alike) : Terminator
  Threshold : quarc_library/Discontinuities/Threshold  operator=>=  param_src=Specify via dialog  threshold=0.5  duration=0.2
      settings: SourceProductName=QUARC Targets
  Triggers (0,1) [4] : Outport  VectorParamsAs1DForOutWhenUnconnected=off
  Joystick Issue (0,1) : Outport  Port=2  VectorParamsAs1DForOutWhenUnconnected=off
  Commands (%) [4] : Outport  Port=3  VectorParamsAs1DForOutWhenUnconnected=off
  wires:
  Host Game Controller/10 -> Terminator2/1
  Pulse Check/1(signal enable) -> Initialization and Conditioning/Enable
  Host Initialize/1 -> Terminator4/1
  FrSKYMapping/6("Arm/Disarm (bool) ") -> Initialization and Conditioning/6(Arm/Disarm (bool))
  Host Initialize/2 -> Terminator1/1
  FrSKYMapping/7(Takeoff/Autoland (bool)) -> Initialization and Conditioning/7(Takeoff/AutoLand (bool))
  Host Game Controller/7 -> Mux/4, FrSKYMapping/6(Rx)
  Host Game Controller/8 -> Mux/5, FrSKYMapping/7(Ry)
  Initialization and Conditioning/3(Commands (%) [4]) -> Commands (%) [4]/1
  Host Game Controller/5 -> Mux/2, FrSKYMapping/4(y)
  Host Game Controller/9 -> Mux/6, FrSKYMapping/8(Rz)
  Host Game Controller/1 -> Pulse Check/1(new)
  Mux/1 -> Compare/1
  Threshold/1 -> NOT/1, Initialization and Conditioning/8(Joystick Issue (bool))
  AND/1 -> Threshold/1
  Host Game Controller/3 -> FrSKYMapping/2(Sliders)
  Threshold/2 -> Terminator/1
  NOT/1 -> FrSKYMapping/Enable
  Constant/1 -> Compare/2
  Host Game Controller/6 -> Mux/3, FrSKYMapping/5(z)
  FrSKYMapping/4(Roll (%)) -> Initialization and Conditioning/4(Roll (%))
  FrSKYMapping/5(Pitch (%)) -> Initialization and Conditioning/5(Pitch (%))
  Compare/1 -> AND/1
  FrSKYMapping/1(Emergency Abort (bool)) -> Initialization and Conditioning/1(Emergency Abort (bool))
  Initialization and Conditioning/1(Joystick Issue (0,1)) -> Joystick Issue (0,1)/1
  Initialization and Conditioning/2(Triggers (0,1) [4]) -> Triggers (0,1) [4]/1
  FrSKYMapping/2(Yaw (%)) -> Initialization and Conditioning/2(Yaw (%))
  Host Game Controller/4 -> Mux/1, FrSKYMapping/3(x)
  Host Game Controller/2 -> FrSKYMapping/1(Buttons)
  FrSKYMapping/3(Throttle (%)) -> Initialization and Conditioning/3(Throttle (%))

== system QD2_MissionCtrl_Swarm_4x_R2021a/MISSION SERVER QDRONE SWARM/JOYSTICK_SPEKTRUM ==
  note: Throttle
      | Roll
      | Pitch
      | Yaw
  Host Game Controller : quarc_library/Devices/Peripherals/Host/Host Game Controller  object_name=Host-2  controller=1  buffer_size=20  deadzone=[]  saturation=[]  sample_time=qc_get_step_size  auto_center=off  enabled=on  debug_mode=off
      settings: SourceProductName=QUARC Targets
  Host Initialize : quarc_library/Devices/Peripherals/Host/Host Initialize  object_name=Host-2  uri_source=Use external mode communications  uri=tcpip://localhost:18001  send_buffer_size=1000  receive_buffer_size=1000  thread_priority=0  run_client=on  use_window=off  window_position=[]  sample_time=qc_get_step_size  active=on
      settings: SourceProductName=QUARC Targets
  Initialization and Conditioning : Subsystem  TreatAsAtomicUnit=on
  Pulse Check : Subsystem  TreatAsAtomicUnit=on
  Spectrum DXe Mapping : Subsystem
  Terminator{1..4} (4 alike) : Terminator
  Triggers (0,1) [4] : Outport  VectorParamsAs1DForOutWhenUnconnected=off
  Joystick Issue (0,1) : Outport  Port=2  VectorParamsAs1DForOutWhenUnconnected=off
  Commands (%) [4] : Outport  Port=3  VectorParamsAs1DForOutWhenUnconnected=off
  wires:
  Pulse Check/1(signal enable) -> Initialization and Conditioning/Enable
  Host Game Controller/1 -> Pulse Check/1(new), Spectrum DXe Mapping/1(new)
  Initialization and Conditioning/3(Commands (%) [4]) -> Commands (%) [4]/1
  Spectrum DXe Mapping/8(Takeoff/Autoland (bool)) -> Initialization and Conditioning/8(Takeoff/AutoLand (bool))
  Initialization and Conditioning/2(Triggers (0,1) [4]) -> Triggers (0,1) [4]/1
  Spectrum DXe Mapping/2(Emergency Abort (bool)) -> Initialization and Conditioning/2(Emergency Abort (bool))
  Host Game Controller/2 -> Spectrum DXe Mapping/2(buttons)
  Spectrum DXe Mapping/6(Pitch (%)) -> Initialization and Conditioning/6(Pitch (%))
  Spectrum DXe Mapping/4(Throttle (%)) -> Initialization and Conditioning/4(Throttle (%))
  Spectrum DXe Mapping/5(Roll (%)) -> Initialization and Conditioning/5(Roll (%))
  Spectrum DXe Mapping/7("Arm/Disarm (bool) ") -> Initialization and Conditioning/7(Arm/Disarm (bool))
  Spectrum DXe Mapping/3(Yaw (%)) -> Initialization and Conditioning/3(Yaw (%))
  Host Initialize/2 -> Terminator1/1
  Host Initialize/1 -> Terminator4/1
  Host Game Controller/6 -> Spectrum DXe Mapping/6(z)
  Host Game Controller/3 -> Spectrum DXe Mapping/3(Sliders)
  Host Game Controller/5 -> Spectrum DXe Mapping/5(y)
  Host Game Controller/4 -> Spectrum DXe Mapping/4(x)
  Host Game Controller/8 -> Spectrum DXe Mapping/8(Ry)
  Host Game Controller/9 -> Terminator2/1
  Host Game Controller/10 -> Terminator3/1
  Host Game Controller/7 -> Spectrum DXe Mapping/7(Rx)
  Spectrum DXe Mapping/1(Joystick Issue (bool)) -> Initialization and Conditioning/1(Joystick Issue (bool))
  Initialization and Conditioning/1(Joystick Issue (0,1)) -> Joystick Issue (0,1)/1
